simulink model "verify_AddSolarPosition_mdl"  (Simulink 8.2)
settings: Solver=FixedStepDiscrete  StartTime=0.0  StopTime=24*3600  FixedStep=3600  RelTol=1e-3
libraries: carnot x2
settings Model: Creator=drhf  LastModifiedBy=drhf

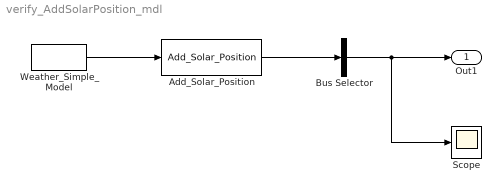
== system verify_AddSolarPosition_mdl ==
  Add_Solar_Position : carnot/Weather/Add_Solar_Position  longi=0  lati=45  timezone=0
  Bus Selector : BusSelector  OutputSignals=Zenith_Angle,Azimuth_Angle  OutputAsBus=on
  Scope : Scope
  Weather_Simple_Model : carnot/Weather/Weather_Simple_Model  lat=45  Ibn=900  Idg=100  tamb=5  deltaTsky=-6  rh=50  precip="10e-3/24/3600           % 10 mm in 24 h"  cloud=0.125  p=1013e2  vw=1  wdir=270
  Out1 : Outport
  wires:
  Add_Solar_Position/1 -> Bus Selector/1
  Weather_Simple_Model/1 -> Add_Solar_Position/1
  Bus Selector/1 -> Out1/1, Scope/1
